simulink model "demoimaqsl_rgbhistogram_maccam"  (R2013b)
settings: Solver=FixedStepDiscrete  StartTime=0.0  StopTime=inf  RelTol=1e-3
undefined symbols (not defined in the file or in its folder): gray, IsPositionTracked, IsSkeletonTracked, JointDepthIndices, JointImageIndices, JointTrackingState, JointWorldCoordinates, M, N, none, PositionDepthIndices, PositionImageIndices, PositionWorldCoordinates, SegmentationData, SkeletonTrackingID, videoinput
libraries: dspstat3 x3, imaqlib x1, dspsnks4 x1, visionsinks x1
settings Model: FPTRunName=Active  Creator=don  LastModifiedBy=koreyk
settings DataIOCC: SignalLoggingSaveFormat=ModelDataLogs  SaveOutput=off  SaveTime=off  SignalLoggingName=sigsOut
settings OptimizationCC: ExpressionDepthLimit=2147483647  InitFltsAndDblsToZero=on
settings DebuggingCC: SaveWithParameterizedLinksMsg=none  CheckExecutionContextPreStartOutputMsg=on  CheckExecutionContextRuntimeOutputMsg=on  SignalResolutionControl=TryResolveAllWithWarning  SolverPrmCheckMsg=none  MultiTaskDSMMsg=warning  MultiTaskCondExecSysMsg=none  FcnCallInpInsideContextMsg=UseLocalSettings  StateNameClashWarn=warning  StrictBusMsg=None
settings HardwareCC: TargetUnknown=on
settings RTWCC: IncludeERTFirstTime=on
settings GRTTargetCC: TargetFcnLib=ansi_tfl_tmw.mat  CombineOutputUpdateFcns=off  GRTInterface=on

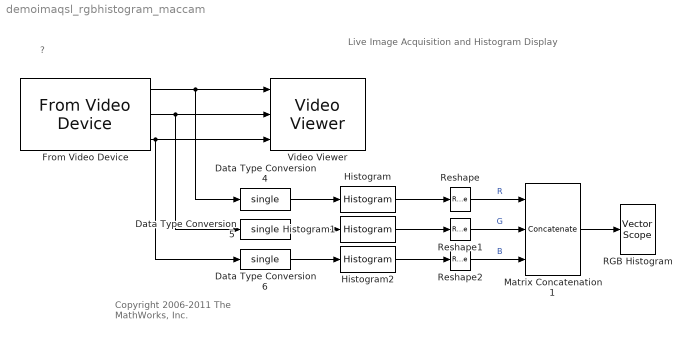
== system demoimaqsl_rgbhistogram_maccam ==
  note: Live Image Acquisition and Histogram Display
  note: ?
  note: Copyright 2006-2011 The MathWorks, Inc.
  Data Type Conversion4 : DataTypeConversion  OutDataTypeStr=single  SaturateOnIntegerOverflow=on  RndMeth=Zero
  Data Type Conversion5 : DataTypeConversion  OutDataTypeStr=single  SaturateOnIntegerOverflow=on  RndMeth=Zero
  Data Type Conversion6 : DataTypeConversion  OutDataTypeStr=single  SaturateOnIntegerOverflow=on  RndMeth=Zero
  From Video Device : imaqlib/From Video Device  DeviceMenu=macvideo 1 (FaceTime Camera (Built-in))  Device=macvideo 1 (FaceTime Camera (Built-in))  ObjConstructor=videoinput('macvideo', 1)  VideoFormatMenu=YCbCr422_640x480  VideoFormat=YCbCr422_640x480  VideoSource=default  ROIPosition=[0 0 480 640]  EnableHWTrigger=off  TriggerConfiguration=none/none  SampleTime=1/30  OutputPortsMode=Separate color signals  DataType=uint8  CanDoHWTrigger=no  ReturnedColorSpace=YCbCr  BlockHandle=53.0016  ROIWidth=640  ROIHeight=480  ROIColumn=0  ROIRow=0  EngXMLPath=/Applications/MATLAB_R2013b.app/toolbox/imaq/imaq/private  DevXMLPath=/Applications/MATLAB_R2013b.app/toolbox/imaq/imaqadaptors/maci64  EngLibPath=/Applications/MATLAB_R2013b.app/toolbox/imaq/imaqblks/imaqmex/maci64  ColorSpace=YCbCr  BayerSensorAlignment=grbg  AllMetadata=IsPositionTracked;IsSkeletonTracked;JointDepthIndices;JointImageIndices;JointTrackingState;JointWorldCoordinates;PositionDepthIndices;PositionImageIndices;PositionWorldCoordinates;SegmentationData;SkeletonTrackingID
  Histogram : dspstat3/Histogram  umin=0  umax=255  nbins=256  normalized=off  run=off  reset=on  trigtype=Non-zero sample  operateOver=Entire input  Dimension=1  colComp=on  roundingMode=Floor  overflowMode=off
  Histogram1 : dspstat3/Histogram  umin=0  umax=255  nbins=256  normalized=off  run=off  reset=on  trigtype=Non-zero sample  operateOver=Entire input  Dimension=1  colComp=on  roundingMode=Floor  overflowMode=off
  Histogram2 : dspstat3/Histogram  umin=0  umax=255  nbins=256  normalized=off  run=off  reset=on  trigtype=Non-zero sample  operateOver=Entire input  Dimension=1  colComp=on  roundingMode=Floor  overflowMode=off
  Matrix Concatenation1 : Concatenate  NumInputs=3  Mode=Multidimensional array  ConcatenateDimension=2
  RGB Histogram : dspsnks4/Vector Scope  ScopeProperties=off  Domain=User-defined  HorizSpan=1  DisplayProperties=off  AxisGrid=on  Memory=off  FrameNumber=off  AxisLegend=on  AxisZoom=on  OpenScopeAtSimStart=on  OpenScopeImmediately=off  FigPos=[478 510 321 220]  AxisProperties=on  XUnits=Hertz  XRange=[0...Fs/2]  InheritXIncr=off  XIncr=1  XLabel=Intensity  XLimit=Auto  XMin=0  XMax=1  XStart=0  YUnits=dB  YLabel=Count  LineProperties=off  LineMarkers=None  LineColors=[1 0 0]|[0 1 0]|[0 0 1]  XAxisParamsVer=6.9
      settings: YMin=0  YMax=1000
  Reshape : Reshape  OutputDimensionality=Column vector (2-D)  OutputDimensions=[M,N]
  Reshape1 : Reshape  OutputDimensionality=Column vector (2-D)  OutputDimensions=[M,N]
  Reshape2 : Reshape  OutputDimensionality=Column vector (2-D)  OutputDimensions=[M,N]
  Video Viewer : visionsinks/Video Viewer  inputType=Obsolete7b  imagePorts=Separate color signals  useColorMap=off  colormapValue=gray(256)  specRange=off  minInputVal=0  maxInputVal=255  FigPos=[182 132 238 191]  AxisZoom=on  trueSizedOnce=on  OpenAtMdlStart=on  DefaultConfigurationName=vipscopes.VideoViewerScopeCfg
  wires:
  From Video Device/3 -> Data Type Conversion6/1, Video Viewer/3
  Matrix Concatenation1/1 -> RGB Histogram/1
  Reshape/1 -> Matrix Concatenation1/1  "R"
  Reshape1/1 -> Matrix Concatenation1/2  "G"
  Reshape2/1 -> Matrix Concatenation1/3  "B"
  From Video Device/1 -> Data Type Conversion4/1, Video Viewer/1
  From Video Device/2 -> Data Type Conversion5/1, Video Viewer/2
  Data Type Conversion4/1 -> Histogram/1
  Data Type Conversion5/1 -> Histogram1/1
  Data Type Conversion6/1 -> Histogram2/1
  Histogram/1 -> Reshape/1
  Histogram1/1 -> Reshape1/1
  Histogram2/1 -> Reshape2/1
